simulink model "zc_detection"  (R2022b)
settings: Solver=ode45  StartTime=0.0  StopTime=10.0  RelTol=1e-3  EnableMultiTasking=on
Description:
  | File Name:  zc_detection
  | 
  | Purpose: Zero Crossing Detection with Saturation, Switch and Abs blocks
  | 
  | Details:
  | 
  | Zero crossing detection is not limited to zero hits in signals. It also
  | applies to sharp edges and corners in signals, as well as the saturation
  | limits of certain block outputs.
  | 
  | If the detection of zero crossings is not significant to a simulation, you
  | can disable it to speed up the simulation. To disable zero crossing
  | control, set the option for Zero crossing control in the Solver pane of the
  | Configuration Parameters dialog to Disable all.
  | 
  | You can see imperfect edges in the simulation results after the option is
  | disabled.
settings Model: Creator=oqaqish  LastModifiedBy=bensweet
settings SolverCC: ZeroCrossControl=EnableAll  AlgebraicLoopSolver=TrustRegion
settings DataIOCC: LimitDataPoints=on  SaveFormat=Array  ReturnWorkspaceOutputs=off  SignalLoggingName=sigsOut
settings OptimizationCC: ExpressionDepthLimit=2147483647  InitFltsAndDblsToZero=on  LifeSpan=inf
settings DebuggingCC: CheckExecutionContextPreStartOutputMsg=on  UnconnectedInputMsg=warning  UnconnectedOutputMsg=warning  UnconnectedLineMsg=warning  PregeneratedLibrarySubsystemCodeDiagnostic=none  SFMachineParentedDataDiag=warning
settings HardwareCC: ProdBitPerPointer=32  ProdBitPerSizeT=32  ProdBitPerPtrDiffT=32  ProdLargestAtomicFloat=None  ProdIntDivRoundTo=Undefined  ProdEndianess=Unspecified  ProdWordSize=32  ProdHWDeviceType=32-bit Generic  TargetUnknown=on
settings ModelReferenceCC: EnableRefExpFcnMdlSchedulingChecks=on  PropagateSignalLabelsOutOfModel=off
settings SFSimCC: SimUseLocalCustomCode=off
settings RTWCC: RTWUseLocalCustomCode=off  DLArmComputeVersion=19.05
settings CodeAppCC: StateflowObjectComments=on
settings GRTTargetCC: TargetFcnLib=ansi_tfl_tmw.mat  TargetLangStandard=C89/C90 (ANSI)  CombineOutputUpdateFcns=off  GRTInterface=on
settings ConfigComp: CovMetricSettings=dw  CovSaveCumulativeToWorkspaceVar=on  CovSaveSingleToWorkspaceVar=on  CovExternalEMLEnable=off  CovSFcnEnable=off

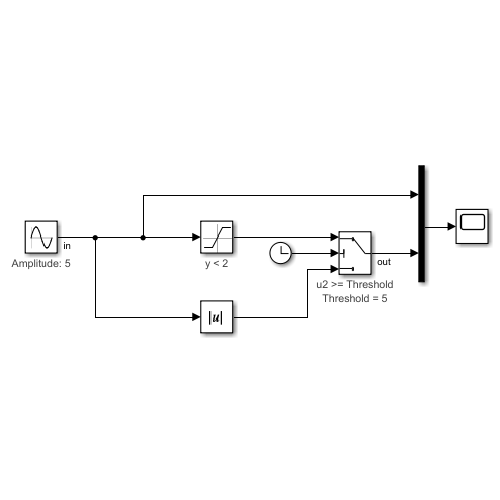
[thumbnail: Simulink's stored preview of the top-level diagram]
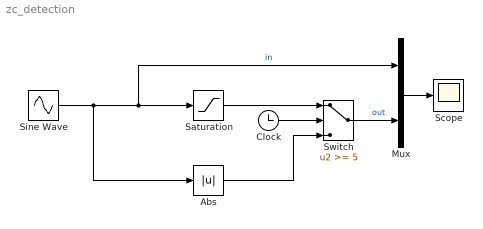
== system zc_detection ==
  Abs : Abs
  Clock : Clock
  Mux : Mux  Inputs=2
  Saturation : Saturate  UpperLimit=2  LowerLimit=-inf
      settings: AttributesFormatString=y < %<UpperLimit>\n
  Scope : Scope
  Sine Wave : Sin  Amplitude=5  SampleTime=0
      settings: AttributesFormatString=Amplitude: %<Amplitude>
  Switch : Switch  Threshold=5  InputSameDT=off
      settings: AttributesFormatString=%<Criteria>\nThreshold = %<Threshold>
  wires:
  Sine Wave/1 -> Abs/1, Saturation/1, Mux/1  "in"
  Mux/1 -> Scope/1
  Switch/1 -> Mux/2  "out"
  Saturation/1 -> Switch/1
  Abs/1 -> Switch/3
  Clock/1 -> Switch/2
